simulink model "canPack_ADC1_EPS_02"  (R2020a)
settings: Solver=VariableStepAuto  StartTime=0.0  StopTime=10.0  RelTol=1e-3
libraries: MyLibrary x1
settings Model: Creator=Administrator  LastModifiedBy=Administrator

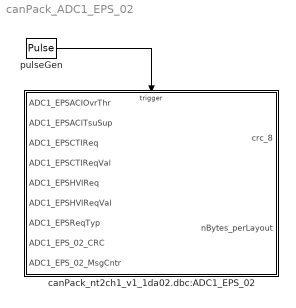
== system canPack_ADC1_EPS_02 ==
  canPack_nt2ch1_v1_1da02.dbc:ADC1_EPS_02 : Subsystem
  pulseGen : DiscretePulseGenerator  PulseType=Time based  Period=0.02  PulseWidth=50
  wires:
  pulseGen/1 -> canPack_nt2ch1_v1_1da02.dbc:ADC1_EPS_02/Trigger

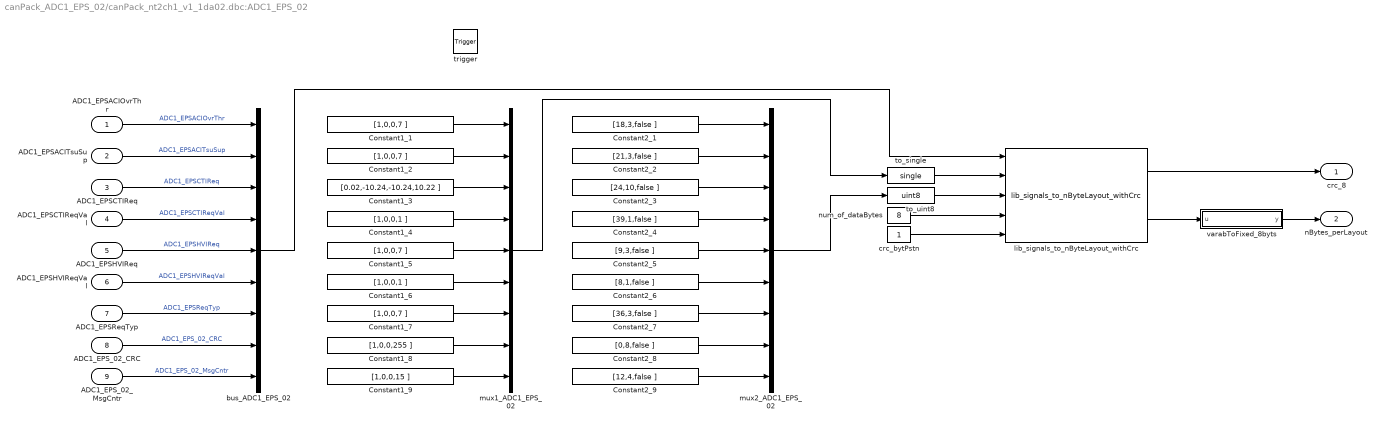
== system canPack_ADC1_EPS_02/canPack_nt2ch1_v1_1da02.dbc:ADC1_EPS_02 ==
  ADC1_EPSACIOvrThr : Inport
  ADC1_EPSACITsuSup : Inport  Port=2
  ADC1_EPSCTIReq : Inport  Port=3
  ADC1_EPSCTIReqVal : Inport  Port=4
  ADC1_EPSHVIReq : Inport  Port=5
  ADC1_EPSHVIReqVal : Inport  Port=6
  ADC1_EPSReqTyp : Inport  Port=7
  ADC1_EPS_02_CRC : Inport  Port=8
  ADC1_EPS_02_MsgCntr : Inport  Port=9
  trigger : TriggerPort  VariantControl=Variant  PortDimensions=1
  Constant1_{1..2,5,7} (4 alike) : Constant  Value=[1,0,0,7 ]  SampleTime=-1
  Constant1_3 : Constant  Value=[0.02,-10.24,-10.24,10.22 ]  SampleTime=-1
  Constant1_4 : Constant  Value=[1,0,0,1 ]  SampleTime=-1
  Constant1_6 : Constant  Value=[1,0,0,1 ]  SampleTime=-1
  Constant1_8 : Constant  Value=[1,0,0,255 ]  SampleTime=-1
  Constant1_9 : Constant  Value=[1,0,0,15 ]  SampleTime=-1
  Constant2_1 : Constant  Value=[18,3,false ]  SampleTime=-1
  Constant2_2 : Constant  Value=[21,3,false ]  SampleTime=-1
  Constant2_3 : Constant  Value=[24,10,false ]  SampleTime=-1
  Constant2_4 : Constant  Value=[39,1,false ]  SampleTime=-1
  Constant2_5 : Constant  Value=[9,3,false ]  SampleTime=-1
  Constant2_6 : Constant  Value=[8,1,false ]  SampleTime=-1
  Constant2_7 : Constant  Value=[36,3,false ]  SampleTime=-1
  Constant2_8 : Constant  Value=[0,8,false ]  SampleTime=-1
  Constant2_9 : Constant  Value=[12,4,false ]  SampleTime=-1
  bus_ADC1_EPS_02 : BusCreator  Inputs=9
  crc_bytPstn : Constant  OutDataTypeStr=uint8  SampleTime=-1
  lib_signals_to_nByteLayout_withCrc : MyLibrary/lib_signals_to_nByteLayout_withCrc  SystemSampleTime=-1  Latency=0  AutoFrameSizeCalculation=off
  mux1_ADC1_EPS_02 : Mux  Inputs=9
  mux2_ADC1_EPS_02 : Mux  Inputs=9
  num_of_dataBytes : Constant  Value=8  OutDataTypeStr=uint8  SampleTime=-1
  to_single : DataTypeConversion  OutDataTypeStr=single
  to_uint8 : DataTypeConversion  OutDataTypeStr=uint8
  varabToFixed_8byts : MATLAB Function  TreatAsAtomicUnit=on
  crc_8 : Outport
  nBytes_perLayout : Outport  Port=2
  wires:
  ADC1_EPSACIOvrThr/1 -> bus_ADC1_EPS_02/1  "ADC1_EPSACIOvrThr"
  ADC1_EPSACITsuSup/1 -> bus_ADC1_EPS_02/2  "ADC1_EPSACITsuSup"
  ADC1_EPSCTIReq/1 -> bus_ADC1_EPS_02/3  "ADC1_EPSCTIReq"
  ADC1_EPSCTIReqVal/1 -> bus_ADC1_EPS_02/4  "ADC1_EPSCTIReqVal"
  ADC1_EPSHVIReq/1 -> bus_ADC1_EPS_02/5  "ADC1_EPSHVIReq"
  ADC1_EPSHVIReqVal/1 -> bus_ADC1_EPS_02/6  "ADC1_EPSHVIReqVal"
  ADC1_EPSReqTyp/1 -> bus_ADC1_EPS_02/7  "ADC1_EPSReqTyp"
  ADC1_EPS_02_CRC/1 -> bus_ADC1_EPS_02/8  "ADC1_EPS_02_CRC"
  ADC1_EPS_02_MsgCntr/1 -> bus_ADC1_EPS_02/9  "ADC1_EPS_02_MsgCntr"
  Constant1_1/1 -> mux1_ADC1_EPS_02/1
  Constant2_1/1 -> mux2_ADC1_EPS_02/1
  Constant1_2/1 -> mux1_ADC1_EPS_02/2
  Constant2_2/1 -> mux2_ADC1_EPS_02/2
  Constant1_3/1 -> mux1_ADC1_EPS_02/3
  Constant2_3/1 -> mux2_ADC1_EPS_02/3
  Constant1_4/1 -> mux1_ADC1_EPS_02/4
  Constant2_4/1 -> mux2_ADC1_EPS_02/4
  Constant1_5/1 -> mux1_ADC1_EPS_02/5
  Constant2_5/1 -> mux2_ADC1_EPS_02/5
  Constant1_6/1 -> mux1_ADC1_EPS_02/6
  Constant2_6/1 -> mux2_ADC1_EPS_02/6
  Constant1_7/1 -> mux1_ADC1_EPS_02/7
  Constant2_7/1 -> mux2_ADC1_EPS_02/7
  Constant1_8/1 -> mux1_ADC1_EPS_02/8
  Constant2_8/1 -> mux2_ADC1_EPS_02/8
  Constant1_9/1 -> mux1_ADC1_EPS_02/9
  Constant2_9/1 -> mux2_ADC1_EPS_02/9
  bus_ADC1_EPS_02/1 -> lib_signals_to_nByteLayout_withCrc/1
  mux1_ADC1_EPS_02/1 -> to_single/1
  to_single/1 -> lib_signals_to_nByteLayout_withCrc/2
  mux2_ADC1_EPS_02/1 -> to_uint8/1
  to_uint8/1 -> lib_signals_to_nByteLayout_withCrc/3
  lib_signals_to_nByteLayout_withCrc/1 -> crc_8/1
  num_of_dataBytes/1 -> lib_signals_to_nByteLayout_withCrc/4
  lib_signals_to_nByteLayout_withCrc/2 -> varabToFixed_8byts/1(u)
  varabToFixed_8byts/1(y) -> nBytes_perLayout/1
  crc_bytPstn/1 -> lib_signals_to_nByteLayout_withCrc/5

== matlab function canPack_ADC1_EPS_02/canPack_nt2ch1_v1_1da02.dbc:ADC1_EPS_02/varabToFixed_8byts ==
  data: u input uint8 size=8; y output uint8
function y = fcn(u)

fixed_size = 8;
y = uint8(zeros(fixed_size,1));

for i=1:fixed_size
    y(i) = u(i);
end
